simulink library "tetherDragForceNGreater2_ul"  (R2018b)
settings: Solver=VariableStepAuto  StartTime=0.0  StopTime=10.0  RelTol=1e-3
values from neighbouring files (symbols this model uses):
  Cd = 0.5    [tetherDragForce_ts.m]
  D = NaN(6*(N-2),1)    [tether_ode.m]
  dia_t = 0.01    [tetherDragForce_ts.m]
  rho_fluid = 1000    [tetherDragForce_ts.m]
settings Model: Creator=asiddiq2  LastModifiedBy=mcobb

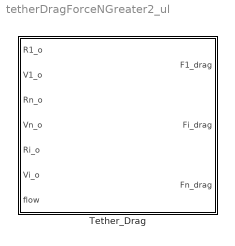
== system tetherDragForceNGreater2_ul ==
  Tether_Drag : Subsystem  mask{N=0, Cd=Cd, rho_fluid=rho_fluid, dia_t=dia_t}
      mask prompts: N "Number of Nodes"; Cd "Drag coefficient"; rho_fluid "Fluid density (kg/m^3)"; dia_t "Tether diameter (m)"

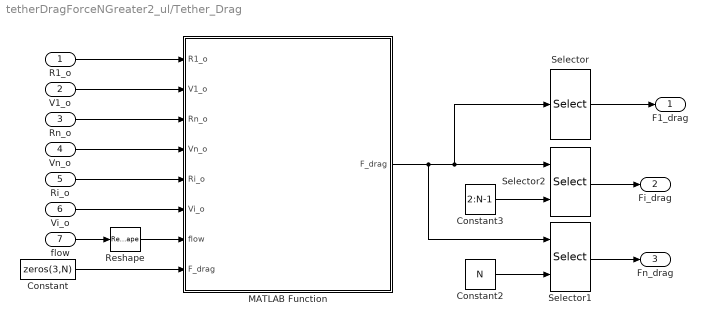
== system tetherDragForceNGreater2_ul/Tether_Drag ==
  R1_o : Inport
  V1_o : Inport  Port=2
  Rn_o : Inport  Port=3
  Vn_o : Inport  Port=4
  Ri_o : Inport  Port=5
  Vi_o : Inport  Port=6
  flow : Inport  Port=7
  Constant : Constant  Value=zeros(3,N)
  Constant2 : Constant  Value=N
  Constant3 : Constant  Value=2:N-1
  MATLAB Function : MATLAB Function  TreatAsAtomicUnit=on
  Reshape : Reshape  OutputDimensionality=Column vector (2-D)
  Selector : Selector  NumberOfDimensions=2  InputPortWidth=3  IndexOptions=Select all,Index vector (dialog)  Indices=[1 3],1  OutputSizes=1,1
  Selector1 : Selector  NumberOfDimensions=2  InputPortWidth=3  IndexOptions=Select all,Index vector (port)  Indices=[1 3],N  OutputSizes=1,1
  Selector2 : Selector  NumberOfDimensions=2  InputPortWidth=3  IndexOptions=Select all,Index vector (port)  Indices=[1 3],[2:N-1]  OutputSizes=1,1
  F1_drag : Outport
  Fi_drag : Outport  Port=2
  Fn_drag : Outport  Port=3
  wires:
  flow/1 -> Reshape/1
  Constant/1 -> MATLAB Function/8("F_drag ")
  Reshape/1 -> MATLAB Function/7(flow)
  Vi_o/1 -> MATLAB Function/6(Vi_o)
  Ri_o/1 -> MATLAB Function/5(Ri_o)
  Vn_o/1 -> MATLAB Function/4(Vn_o)
  Rn_o/1 -> MATLAB Function/3(Rn_o)
  V1_o/1 -> MATLAB Function/2(V1_o)
  R1_o/1 -> MATLAB Function/1(R1_o)
  Constant3/1 -> Selector2/2
  Constant2/1 -> Selector1/2
  MATLAB Function/1(F_drag) -> Selector/1, Selector2/1, Selector1/1
  Selector/1 -> F1_drag/1
  Selector2/1 -> Fi_drag/1
  Selector1/1 -> Fn_drag/1

== matlab function tetherDragForceNGreater2_ul/Tether_Drag/MATLAB Function ==
  data: R1_o input; V1_o input; Rn_o input; Vn_o input; Ri_o input; F_drag output; Vi_o input; flow input; F_drag input; Cd parameter; dia_t parameter; rho_fluid parameter; N parameter
function F_drag = fcn(R1_o,V1_o,Rn_o,Vn_o,Ri_o,Vi_o,flow,F_drag,Cd, dia_t, rho_fluid, N)

Ri_o = [R1_o Ri_o Rn_o];
Vi_o = [V1_o Vi_o Vn_o];

Ve = zeros(3,N-1);
Vrel = zeros(3,N-1);
drag_direction = zeros(3,N-1);
drag = zeros(3,N-1);

qe = zeros(N-1,1);
di = zeros(N-1,1);
th = zeros(N-1,1);
S = zeros(N-1,1);

% elemental velocity
for i = 1:N-1
    
    % relative velocity
    Ve(:,i) = (Vi_o(:,i) + Vi_o(:,i+1))/2;
    Vrel(:,i) = flow - Ve(:,i);
    Vrel(3,i) = 0;
    % drag direction
    if norm(Vrel(:,i)) > 1e-3
        drag_direction(:,i) = Vrel(:,i)/norm(Vrel(:,i));
    else
        drag_direction(:,i) = zeros(3,1);
    end
    
    % dynamic pressure
    qe(i) = 0.5*rho_fluid*norm(Vrel(:,i))^2;
    
    % projected area
    di(i) = norm(Ri_o(:,i+1)-Ri_o(:,i));
    th(i) = atan( (Ri_o(3,i+1)-Ri_o(3,i))/norm(Ri_o(1:2,i+1)-Ri_o(1:2,i)) );
    S(i) = di(i)*dia_t*sin(th(i));
    
    drag(:,i) = 0.5*rho_fluid*Cd*Vrel(:,i)*norm(Vrel(:,i))*S(i);
end

% drag force acting on each node'
for i = 1:N
    if i == 1
        F_drag(:,i) = drag(:,i)/2;
    elseif i> 1 && i < N
        F_drag(:,i) = (drag(:,i-1) + drag(:,i))/2;
    elseif i == N
        F_drag(:,i) = drag(:,i-1)/2;
    end
end

end
